simulink model "rmd_power_pack_model"  (R2024a)
settings: Solver=FixedStepAuto  StartTime=0.0  StopTime=10.0  RelTol=1e-3
undefined symbols (not defined in the file): cstCurrSensAmplInpRstn, cstMotorMdlSampTime, cstSpicInvtMdlSampTime, DiscIntNeverNeededParam
libraries: nesl_utility x13, simulink x3, fl_lib x2
(part 1 of 2)
settings Model: DataDictionary=dd_power_pack.sldd  EnableAccessToBaseWorkspace=off  Creator=pav2ofo  LastModifiedBy=pav2ofo

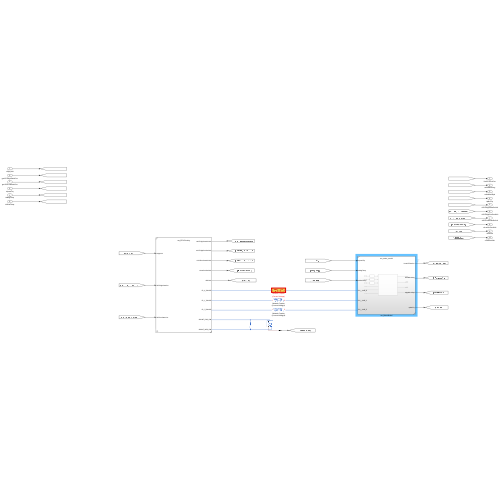
[thumbnail: Simulink's stored preview of the top-level diagram]
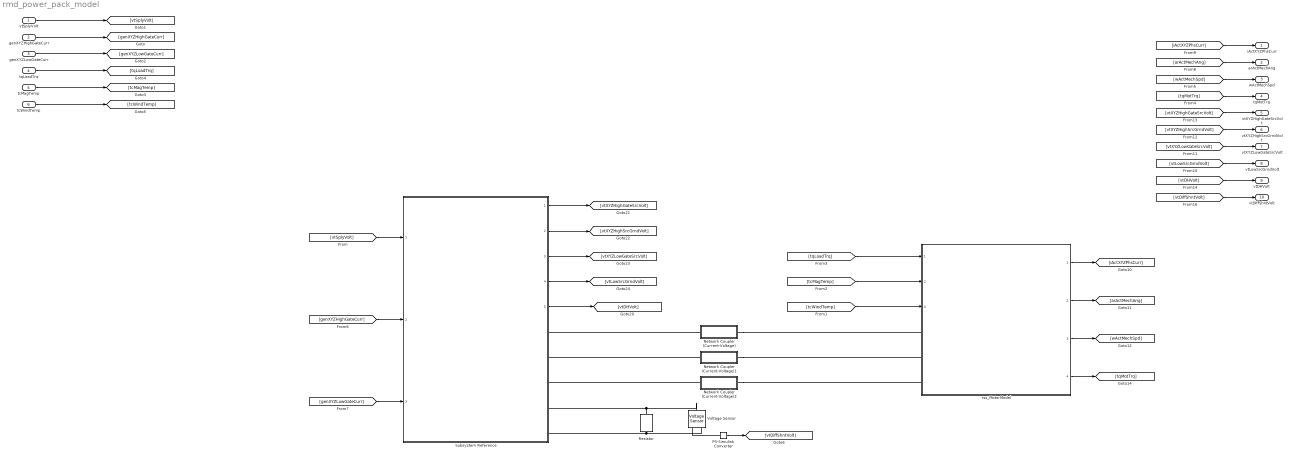
== system rmd_power_pack_model ==
  vtSplyVolt : Inport
  genXYZHighGateCurr : Inport  Port=2
  genXYZLowGateCurr : Inport  Port=3
  tqLoadTrq : Inport  Port=4
  tcMagTemp : Inport  Port=5
  tcWindTemp : Inport  Port=6
  Network Coupler (Current-Voltage) : Subsystem  mask(Network Coupler (Current-Voltage)){}
      mask init:
      | % Icon
      | key = 'Simscape.NetworkCouplers.ElectricalCurrentVoltage';
      | foundation.internal.couplers.updateIcon(gcb,'currentVoltageSource.svg',key)
      settings: OpenFcn=open_system(gcbh,'force')
      mask Help: web([docroot '/simscape/ref/networkcouplercurrentvoltage.html'])
      mask Display:
      | color('red');
      | port_label('LConn', 1,'1')
      | port_label('RConn', 1,'2')
  Network Coupler (Current-Voltage)1 : Subsystem  mask(Network Coupler (Current-Voltage)){}
      mask init:
      | % Icon
      | key = 'Simscape.NetworkCouplers.ElectricalCurrentVoltage';
      | foundation.internal.couplers.updateIcon(gcb,'currentVoltageSource.svg',key)
      settings: OpenFcn=open_system(gcbh,'force')
      mask Help: web([docroot '/simscape/ref/networkcouplercurrentvoltage.html'])
      mask Display:
      | color('red');
      | port_label('LConn', 1,'1')
      | port_label('RConn', 1,'2')
  Network Coupler (Current-Voltage)2 : Subsystem  mask(Network Coupler (Current-Voltage)){}
      mask init:
      | % Icon
      | key = 'Simscape.NetworkCouplers.ElectricalCurrentVoltage';
      | foundation.internal.couplers.updateIcon(gcb,'currentVoltageSource.svg',key)
      settings: OpenFcn=open_system(gcbh,'force')
      mask Help: web([docroot '/simscape/ref/networkcouplercurrentvoltage.html'])
      mask Display:
      | color('red');
      | port_label('LConn', 1,'1')
      | port_label('RConn', 1,'2')
  PS-Simulink Converter : nesl_utility/PS-Simulink Converter  PhysicalDomain=network_engine_domain  SubClassName=ps_output  LeftPortType=input  RightPortType=output  PseudoPeriodic=off  Frequencies=[]  VectorFormat=inherit  Unit=inherit  AffineConversion=off
  Resistor : fl_lib/Electrical/Electrical Elements/Resistor  R=cstCurrSensAmplInpRstn Ohm  i_specify=off  i_priority=None  i=0 A  i_nominal_specify=off  i_nominal_value=1  i_nominal_unit=A  v_specify=off  v_priority=None  v=0 V  v_nominal_specify=off  v_nominal_value=1  v_nominal_unit=V
  Subsystem Reference : Subsystem  SystemSampleTime=cstSpicInvtMdlSampTime  ReferencedSubsystem=rss_ECUCircuitry
  Voltage Sensor : fl_lib/Electrical/Electrical Sensors/Voltage Sensor
  rss_MotorModel : Subsystem  ReferencedSubsystem=rss_motor_model
  iActXYZPhsCurr : Outport
  arActMechAng : Outport  Port=2
  wActMechSpd : Outport  Port=3
  tqMotTrq : Outport  Port=4
  vtXYZHighGateSrcVolt : Outport  Port=5
  vtXYZHighSrcGrndVolt : Outport  Port=6
  vtXYZLowGateSrcVolt : Outport  Port=7
  vtLowSrcGrndVolt : Outport  Port=8
  vtDHVolt : Outport  Port=9
  vtDiffShntVolt : Outport  Port=10
  wires:
  Subsystem Reference/2 -> [vtXYZHighSrcGrndVolt]
  Subsystem Reference/4 -> [vtLowSrcGrndVolt]
  Subsystem Reference/5 -> [vtDHVolt]
  [vtSplyVolt] -> Subsystem Reference/1
  Subsystem Reference/1 -> [vtXYZHighGateSrcVolt]
  Subsystem Reference/3 -> [vtXYZLowGateSrcVolt]
  [genXYZLowGateCurr] -> Subsystem Reference/3
  [tcWindTemp] -> rss_MotorModel/3
  [genXYZHighGateCurr] -> Subsystem Reference/2
  [tqLoadTrq] -> rss_MotorModel/1
  rss_MotorModel/2 -> [arActMechAng]
  rss_MotorModel/4 -> [tqMotTrq]
  rss_MotorModel/3 -> [wActMechSpd]
  rss_MotorModel/1 -> [iActXYZPhsCurr]
  [tcMagTemp] -> rss_MotorModel/2
  vtSplyVolt/1 -> [vtSplyVolt]
  genXYZHighGateCurr/1 -> [genXYZHighGateCurr]
  genXYZLowGateCurr/1 -> [genXYZLowGateCurr]
  tcMagTemp/1 -> [tcMagTemp]
  tcWindTemp/1 -> [tcWindTemp]
  tqLoadTrq/1 -> [tqLoadTrq]
  [arActMechAng] -> arActMechAng/1
  [iActXYZPhsCurr] -> iActXYZPhsCurr/1
  [tqMotTrq] -> tqMotTrq/1
  [wActMechSpd] -> wActMechSpd/1
  [vtXYZLowGateSrcVolt] -> vtXYZLowGateSrcVolt/1
  [vtLowSrcGrndVolt] -> vtLowSrcGrndVolt/1
  [vtXYZHighSrcGrndVolt] -> vtXYZHighSrcGrndVolt/1
  [vtXYZHighGateSrcVolt] -> vtXYZHighGateSrcVolt/1
  [vtDHVolt] -> vtDHVolt/1
  [vtDiffShntVolt] -> vtDiffShntVolt/1
  PS-Simulink Converter/1 -> [vtDiffShntVolt]
  connections:
  Network Coupler (Current-Voltage)1/LConn1 -- Subsystem Reference/RConn2
  Network Coupler (Current-Voltage)/LConn1 -- Subsystem Reference/RConn1
  Network Coupler (Current-Voltage)2/LConn1 -- Subsystem Reference/RConn3
  Network Coupler (Current-Voltage)1/RConn1 -- rss_MotorModel/LConn2
  Network Coupler (Current-Voltage)/RConn1 -- rss_MotorModel/LConn1
  Network Coupler (Current-Voltage)2/RConn1 -- rss_MotorModel/LConn3
  Voltage Sensor/RConn2 -- Resistor/RConn1 -- Subsystem Reference/RConn5
  Resistor/LConn1 -- Voltage Sensor/LConn1 -- Subsystem Reference/RConn4
  PS-Simulink Converter/LConn1 -- Voltage Sensor/RConn1

== system rmd_power_pack_model/Network Coupler (Current-Voltage) ==
  note: Connect Port 1 to the network
      | with the smaller sample time, or
      | the network running variable step.
  note: Uncomment rate transition
      | blocks if one or both networks
      | are running fixed step.
  Port 1 Interface : Subsystem  mask(Network Coupler (Current-Voltage) Port 1 Interface){isThreePhase=off, numNodes=1, samplingType=Fixed step both ports with faster sampling at port 1, ts=1e-3, h1=cstSpicInvtMdlSampTime, h2=cstMotorMdlSampTime, predictionDiscreteToContinuous=off, smoothingContinuousToDiscrete=off, predictionSlowToFast=off, smoothingFastToSlow=off, nSmooth=1, tsSmoothing=0.01, tsMax=0.005, tau=0.001, i0=0, v0=0}
      mask prompts: isThreePhase "physmod:simscape:couplers:SimscapeNetworkCouplersLib:ElectricalThreePhase_MP"; numNodes "physmod:simscape:couplers:SimscapeNetworkCouplersLib:ElectricalNodeArraySize_MP"; samplingType "physmod:simscape:couplers:SimscapeNetworkCouplersLib:SamplingType_MP"; ts "physmod:simscape:couplers:SimscapeNetworkCouplersLib:SeparatorTimeConstants_MP"; h1 "physmod:simscape:couplers:SimscapeNetworkCouplersLib:Port1NetworkDiscreteSampleTimes_MP"; h2 "physmod:simscape:couplers:SimscapeNetworkCouplersLib:Port2NetworkDiscreteSampleTimes_MP"; predictionDiscreteToContinuous "physmod:simscape:couplers:SimscapeNetworkCouplersLib:UsePredictionWhenConnectingFixedStepToVariableStep_MP"; smoothingContinuousToDiscrete "physmod:simscape:couplers:SimscapeNetworkCouplersLib:UseSmoothingWhenConnectingVariableStepToFixedStep_MP"; predictionSlowToFast "physmod:simscape:couplers:SimscapeNetworkCouplersLib:UsePredictionWhenConnectingSlowToFastSampleTimes_MP"; smoothingFastToSlow "physmod:simscape:couplers:SimscapeNetworkCouplersLib:UseSmoothingWhenConnectingFastToSlowSampleTimes_MP"; nSmooth "physmod:simscape:couplers:SimscapeNetworkCouplersLib:NumberOfSamplesOverWhichToSmooth_MP"; tsSmoothing "physmod:simscape:couplers:SimscapeNetworkCouplersLib:SmoothingTimeConstants_MP"; tsMax "physmod:simscape:couplers:SimscapeNetworkCouplersLib:CalculatedFastestTrackableTimeConstants_MP"; tau "physmod:simscape:couplers:SimscapeNetworkCouplersLib:CalculatedFilterTimeConstants_MP"; i0 "physmod:simscape:couplers:SimscapeNetworkCouplersLib:InitialCurrentA_MP"; v0 "physmod:simscape:couplers:SimscapeNetworkCouplersLib:InitialVoltageV_MP"
      mask help: physmod:simscape:couplers:SimscapeNetworkCouplersLib:NetworkCouplerCurrentVoltagePort1Interface_MD
      mask init:
      | % Fixed step sample time value check
      | foundation.internal.couplers.checkSampleTimes(gcb,h1,h2);
      | 
      | % Parameter value checks
      | foundation.internal.couplers.electrical.checkParametersSources(isThreePhase,numNodes,v0,i0);
      | 
      | % Derived parameters
      | [tau,tsMax] = foundation.internal.couplers.electrical.derivedParamsSources(gcb,ts,h1,h2);
      settings: PortSchema="{\"entries\":[{\"content\":{\"sides\":[{\"content\":{\"connectorIds\":[\"LConn1\"]},\"type\":\"ConnectorPlacement.EquallySpacedRectSide\",\"uuid\":\"a6d4a9fd-b5aa-40dc-ab7e-2b646b9b57bc\"},{\"content\":{\"connectorIds\":[\"Out1\",\"In1\"],\"side\":\"RIGHT\"},\"type\":\"ConnectorPlacement.EquallySpacedRectSide\",\"uuid\":\"31bb6273-5b9b-48d0-a1a2-6fbacb979b97\"},{\"content\":{\"connectorIds\":[],\"side\":\"TOP\"},\"type\":\"ConnectorPlacement.EquallySpacedRectSide\",\"uuid\":\"0f7afab2-4481-486c-9ad0-2b42c5b091a4\"}]},\"type\":\"ConnectorPlacement.EquallySpacedConnector\",\"uuid\":\"a98e47aa-cbfd-441a-b14c-c9ea515c056e\"}],\"packageUris\":[\"http://schema.mathworks.com/mf0/Connector/R2020b\"],\"version\":\"1.0\"}"
      mask Help: web([docroot '/simscape/ref/networkcouplercurrentvoltage.html'])
      mask Callback isThreePhase: foundation.internal.couplers.electrical.parameterVisibilitiesThreePhase(gcb)
      mask TypeOptions samplingType: physmod:simscape:couplers:SimscapeNetworkCouplersLib:VariableStepAtPorts1And2_PV | physmod:simscape:couplers:SimscapeNetworkCouplersLib:VariableStepAtPort1AndFixedStepAtPort2_PV | physmod:simscape:couplers:SimscapeNetworkCouplersLib:FixedStepBothPortsWithCommonSampleTime_PV | physmod:simscape:couplers:SimscapeNetworkCouplersLib:FixedStepBothPortsWithFasterSamplingAtPort1_PV
      mask Callback samplingType: foundation.internal.couplers.electrical.parameterVisibilitiesSources(gcb)
      mask Callback predictionDiscreteToContinuous: foundation.internal.couplers.electrical.parameterVisibilitiesSources(gcb)
      mask Callback smoothingContinuousToDiscrete: foundation.internal.couplers.electrical.parameterVisibilitiesSources(gcb)
      mask Callback predictionSlowToFast: foundation.internal.couplers.electrical.parameterVisibilitiesSources(gcb)
      mask Callback smoothingFastToSlow: foundation.internal.couplers.electrical.parameterVisibilitiesSources(gcb)
      mask DialogControl Main Prompt: physmod:simscape:couplers:SimscapeNetworkCouplersLib:tab_Main
      mask DialogControl isThreePhase Prompt: Use three-phase electrical connections
      mask DialogControl numNodes Prompt: Electrical node array size
      mask DialogControl samplingType Prompt: Sampling type
      mask DialogControl ts Prompt: Separator time constant (s)
      mask DialogControl h1 Prompt: Port 1 network discrete sample time (s)
      mask DialogControl h2 Prompt: Port 2 network discrete sample time (s)
      mask DialogControl predictionDiscreteToContinuous Prompt: Use prediction when connecting fixed step to variable step
      mask DialogControl smoothingContinuousToDiscrete Prompt: Use smoothing when connecting variable step to fixed step
      mask DialogControl predictionSlowToFast Prompt: Use prediction when connecting slow to fast sample times
      mask DialogControl smoothingFastToSlow Prompt: Use smoothing when connecting fast to slow sample times
      mask DialogControl nSmooth Prompt: Number of samples over which to smooth
      mask DialogControl tsSmoothing Prompt: Smoothing time constant (s)
      mask DialogControl Analysis Prompt: physmod:simscape:couplers:SimscapeNetworkCouplersLib:tab_Analysis
      mask DialogControl tsMax Prompt: Calculated fastest trackable time constant (s)
      mask DialogControl tau Prompt: Calculated filter time constant (s)
      mask DialogControl updateRecommendations Prompt: physmod:simscape:couplers:SimscapeNetworkCouplersLib:button_Update
      mask DialogControl updateRecommendations Callback: foundation.internal.couplers.electrical.analysisSources(gcb);
      mask DialogControl InitialConditions Prompt: physmod:simscape:couplers:SimscapeNetworkCouplersLib:tab_InitialConditions
      mask DialogControl i0 Prompt: Initial current (A)
      mask DialogControl v0 Prompt: Initial voltage (V)
  Port 2 Interface : Subsystem  mask(Network Coupler (Current-Voltage) Port 2 Interface){isThreePhase=off, numNodes=1}
      mask prompts: isThreePhase "physmod:simscape:couplers:SimscapeNetworkCouplersLib:ElectricalThreePhase_MP"; numNodes "physmod:simscape:couplers:SimscapeNetworkCouplersLib:ElectricalNodeArraySize_MP"
      mask help: physmod:simscape:couplers:SimscapeNetworkCouplersLib:NetworkCouplerCurrentVoltagePort2Interface_MD
      mask init:
      | % Parameter value checks
      | foundation.internal.couplers.electrical.checkParametersNumNodes(isThreePhase,numNodes);
      settings: PortSchema="{\"entries\":[{\"content\":{\"sides\":[{\"content\":{\"connectorIds\":[\"In1\",\"Out1\"]},\"type\":\"ConnectorPlacement.EquallySpacedRectSide\",\"uuid\":\"5a4c1550-e77d-42df-bf3e-b81963920de7\"},{\"content\":{\"connectorIds\":[\"RConn1\"],\"side\":\"RIGHT\"},\"type\":\"ConnectorPlacement.EquallySpacedRectSide\",\"uuid\":\"3fd730f7-5937-4563-a365-595aaae9027b\"},{\"content\":{\"connectorIds\":[],\"side\":\"TOP\"},\"type\":\"ConnectorPlacement.EquallySpacedRectSide\",\"uuid\":\"c16e04e4-26e8-4fd6-98d3-59adbef44c0d\"}]},\"type\":\"ConnectorPlacement.EquallySpacedConnector\",\"uuid\":\"5588d8d0-d459-45fe-a303-1ca6654e99d0\"}],\"packageUris\":[\"http://schema.mathworks.com/mf0/Connector/R2020b\"],\"version\":\"1.0\"}"
      mask Help: web([docroot '/simscape/ref/networkcouplercurrentvoltage.html'])
      mask Callback isThreePhase: foundation.internal.couplers.electrical.parameterVisibilitiesThreePhase(gcb)
      mask DialogControl isThreePhase Prompt: Use three-phase electrical connections
      mask DialogControl numNodes Prompt: Electrical node array size
  Rate transition (fast-to-slow) : RateTransition  Commented=through  Integrity=off
  Rate transition (slow-to-fast) : RateTransition  Commented=through  Integrity=off
  1 : PMIOPort  Side=Left
  2 : PMIOPort  Port=2  Side=Right
  wires:
  Rate transition (slow-to-fast)/1 -> Port 1 Interface/1(current)
  Port 2 Interface/1(current) -> Rate transition (slow-to-fast)/1
  Rate transition (fast-to-slow)/1 -> Port 2 Interface/1(voltage)
  Port 1 Interface/1(voltage) -> Rate transition (fast-to-slow)/1
  connections:
  1/RConn1 -- Port 1 Interface/LConn1
  2/RConn1 -- Port 2 Interface/RConn1

== system rmd_power_pack_model/Network Coupler (Current-Voltage)1 ==
  note: Uncomment rate transition
      | blocks if one or both networks
      | are running fixed step.
  note: Connect Port 1 to the network
      | with the smaller sample time, or
      | the network running variable step.
  Port 1 Interface : Subsystem  mask(Network Coupler (Current-Voltage) Port 1 Interface){isThreePhase=off, numNodes=1, samplingType=Fixed step both ports with faster sampling at port 1, ts=1e-3, h1=10e-9, h2=62.5e-6, predictionDiscreteToContinuous=off, smoothingContinuousToDiscrete=off, predictionSlowToFast=off, smoothingFastToSlow=off, nSmooth=1, tsSmoothing=0.01, tsMax=0.005, tau=0.001, i0=0, v0=0}
      mask prompts: isThreePhase "physmod:simscape:couplers:SimscapeNetworkCouplersLib:ElectricalThreePhase_MP"; numNodes "physmod:simscape:couplers:SimscapeNetworkCouplersLib:ElectricalNodeArraySize_MP"; samplingType "physmod:simscape:couplers:SimscapeNetworkCouplersLib:SamplingType_MP"; ts "physmod:simscape:couplers:SimscapeNetworkCouplersLib:SeparatorTimeConstants_MP"; h1 "physmod:simscape:couplers:SimscapeNetworkCouplersLib:Port1NetworkDiscreteSampleTimes_MP"; h2 "physmod:simscape:couplers:SimscapeNetworkCouplersLib:Port2NetworkDiscreteSampleTimes_MP"; predictionDiscreteToContinuous "physmod:simscape:couplers:SimscapeNetworkCouplersLib:UsePredictionWhenConnectingFixedStepToVariableStep_MP"; smoothingContinuousToDiscrete "physmod:simscape:couplers:SimscapeNetworkCouplersLib:UseSmoothingWhenConnectingVariableStepToFixedStep_MP"; predictionSlowToFast "physmod:simscape:couplers:SimscapeNetworkCouplersLib:UsePredictionWhenConnectingSlowToFastSampleTimes_MP"; smoothingFastToSlow "physmod:simscape:couplers:SimscapeNetworkCouplersLib:UseSmoothingWhenConnectingFastToSlowSampleTimes_MP"; nSmooth "physmod:simscape:couplers:SimscapeNetworkCouplersLib:NumberOfSamplesOverWhichToSmooth_MP"; tsSmoothing "physmod:simscape:couplers:SimscapeNetworkCouplersLib:SmoothingTimeConstants_MP"; tsMax "physmod:simscape:couplers:SimscapeNetworkCouplersLib:CalculatedFastestTrackableTimeConstants_MP"; tau "physmod:simscape:couplers:SimscapeNetworkCouplersLib:CalculatedFilterTimeConstants_MP"; i0 "physmod:simscape:couplers:SimscapeNetworkCouplersLib:InitialCurrentA_MP"; v0 "physmod:simscape:couplers:SimscapeNetworkCouplersLib:InitialVoltageV_MP"
      mask help: physmod:simscape:couplers:SimscapeNetworkCouplersLib:NetworkCouplerCurrentVoltagePort1Interface_MD
      mask init: same as rmd_power_pack_model/Network Coupler (Current-Voltage)/Port 1 Interface
      settings: PortSchema="{\"entries\":[{\"content\":{\"sides\":[{\"content\":{\"connectorIds\":[\"LConn1\"]},\"type\":\"ConnectorPlacement.EquallySpacedRectSide\",\"uuid\":\"a6d4a9fd-b5aa-40dc-ab7e-2b646b9b57bc\"},{\"content\":{\"connectorIds\":[\"Out1\",\"In1\"],\"side\":\"RIGHT\"},\"type\":\"ConnectorPlacement.EquallySpacedRectSide\",\"uuid\":\"31bb6273-5b9b-48d0-a1a2-6fbacb979b97\"},{\"content\":{\"connectorIds\":[],\"side\":\"TOP\"},\"type\":\"ConnectorPlacement.EquallySpacedRectSide\",\"uuid\":\"0f7afab2-4481-486c-9ad0-2b42c5b091a4\"}]},\"type\":\"ConnectorPlacement.EquallySpacedConnector\",\"uuid\":\"a98e47aa-cbfd-441a-b14c-c9ea515c056e\"}],\"packageUris\":[\"http://schema.mathworks.com/mf0/Connector/R2020b\"],\"version\":\"1.0\"}"
      mask Help: web([docroot '/simscape/ref/networkcouplercurrentvoltage.html'])
      mask Callback isThreePhase: foundation.internal.couplers.electrical.parameterVisibilitiesThreePhase(gcb)
      mask TypeOptions samplingType: physmod:simscape:couplers:SimscapeNetworkCouplersLib:VariableStepAtPorts1And2_PV | physmod:simscape:couplers:SimscapeNetworkCouplersLib:VariableStepAtPort1AndFixedStepAtPort2_PV | physmod:simscape:couplers:SimscapeNetworkCouplersLib:FixedStepBothPortsWithCommonSampleTime_PV | physmod:simscape:couplers:SimscapeNetworkCouplersLib:FixedStepBothPortsWithFasterSamplingAtPort1_PV
      mask Callback samplingType: foundation.internal.couplers.electrical.parameterVisibilitiesSources(gcb)
      mask Callback predictionDiscreteToContinuous: foundation.internal.couplers.electrical.parameterVisibilitiesSources(gcb)
      mask Callback smoothingContinuousToDiscrete: foundation.internal.couplers.electrical.parameterVisibilitiesSources(gcb)
      mask Callback predictionSlowToFast: foundation.internal.couplers.electrical.parameterVisibilitiesSources(gcb)
      mask Callback smoothingFastToSlow: foundation.internal.couplers.electrical.parameterVisibilitiesSources(gcb)
      mask DialogControl Main Prompt: physmod:simscape:couplers:SimscapeNetworkCouplersLib:tab_Main
      mask DialogControl isThreePhase Prompt: Use three-phase electrical connections
      mask DialogControl numNodes Prompt: Electrical node array size
      mask DialogControl samplingType Prompt: Sampling type
      mask DialogControl ts Prompt: Separator time constant (s)
      mask DialogControl h1 Prompt: Port 1 network discrete sample time (s)
      mask DialogControl h2 Prompt: Port 2 network discrete sample time (s)
      mask DialogControl predictionDiscreteToContinuous Prompt: Use prediction when connecting fixed step to variable step
      mask DialogControl smoothingContinuousToDiscrete Prompt: Use smoothing when connecting variable step to fixed step
      mask DialogControl predictionSlowToFast Prompt: Use prediction when connecting slow to fast sample times
      mask DialogControl smoothingFastToSlow Prompt: Use smoothing when connecting fast to slow sample times
      mask DialogControl nSmooth Prompt: Number of samples over which to smooth
      mask DialogControl tsSmoothing Prompt: Smoothing time constant (s)
      mask DialogControl Analysis Prompt: physmod:simscape:couplers:SimscapeNetworkCouplersLib:tab_Analysis
      mask DialogControl tsMax Prompt: Calculated fastest trackable time constant (s)
      mask DialogControl tau Prompt: Calculated filter time constant (s)
      mask DialogControl updateRecommendations Prompt: physmod:simscape:couplers:SimscapeNetworkCouplersLib:button_Update
      mask DialogControl updateRecommendations Callback: foundation.internal.couplers.electrical.analysisSources(gcb);
      mask DialogControl InitialConditions Prompt: physmod:simscape:couplers:SimscapeNetworkCouplersLib:tab_InitialConditions
      mask DialogControl i0 Prompt: Initial current (A)
      mask DialogControl v0 Prompt: Initial voltage (V)
  Port 2 Interface : Subsystem  mask(Network Coupler (Current-Voltage) Port 2 Interface){isThreePhase=off, numNodes=1}
      mask prompts: isThreePhase "physmod:simscape:couplers:SimscapeNetworkCouplersLib:ElectricalThreePhase_MP"; numNodes "physmod:simscape:couplers:SimscapeNetworkCouplersLib:ElectricalNodeArraySize_MP"
      mask help: physmod:simscape:couplers:SimscapeNetworkCouplersLib:NetworkCouplerCurrentVoltagePort2Interface_MD
      mask init:
      | % Parameter value checks
      | foundation.internal.couplers.electrical.checkParametersNumNodes(isThreePhase,numNodes);
      settings: PortSchema="{\"entries\":[{\"content\":{\"sides\":[{\"content\":{\"connectorIds\":[\"In1\",\"Out1\"]},\"type\":\"ConnectorPlacement.EquallySpacedRectSide\",\"uuid\":\"5a4c1550-e77d-42df-bf3e-b81963920de7\"},{\"content\":{\"connectorIds\":[\"RConn1\"],\"side\":\"RIGHT\"},\"type\":\"ConnectorPlacement.EquallySpacedRectSide\",\"uuid\":\"3fd730f7-5937-4563-a365-595aaae9027b\"},{\"content\":{\"connectorIds\":[],\"side\":\"TOP\"},\"type\":\"ConnectorPlacement.EquallySpacedRectSide\",\"uuid\":\"c16e04e4-26e8-4fd6-98d3-59adbef44c0d\"}]},\"type\":\"ConnectorPlacement.EquallySpacedConnector\",\"uuid\":\"5588d8d0-d459-45fe-a303-1ca6654e99d0\"}],\"packageUris\":[\"http://schema.mathworks.com/mf0/Connector/R2020b\"],\"version\":\"1.0\"}"
      mask Help: web([docroot '/simscape/ref/networkcouplercurrentvoltage.html'])
      mask Callback isThreePhase: foundation.internal.couplers.electrical.parameterVisibilitiesThreePhase(gcb)
      mask DialogControl isThreePhase Prompt: Use three-phase electrical connections
      mask DialogControl numNodes Prompt: Electrical node array size
  Rate transition (fast-to-slow) : RateTransition  Commented=through  Integrity=off
  Rate transition (slow-to-fast) : RateTransition  Commented=through  Integrity=off
  1 : PMIOPort  Side=Left
  2 : PMIOPort  Port=2  Side=Right
  wires:
  Port 1 Interface/1(voltage) -> Rate transition (fast-to-slow)/1
  Rate transition (fast-to-slow)/1 -> Port 2 Interface/1(voltage)
  Port 2 Interface/1(current) -> Rate transition (slow-to-fast)/1
  Rate transition (slow-to-fast)/1 -> Port 1 Interface/1(current)
  connections:
  2/RConn1 -- Port 2 Interface/RConn1
  1/RConn1 -- Port 1 Interface/LConn1

== system rmd_power_pack_model/Network Coupler (Current-Voltage)2 ==
  note: Connect Port 1 to the network
      | with the smaller sample time, or
      | the network running variable step.
  note: Uncomment rate transition
      | blocks if one or both networks
      | are running fixed step.
  Port 1 Interface : Subsystem  mask(Network Coupler (Current-Voltage) Port 1 Interface){isThreePhase=off, numNodes=1, samplingType=Fixed step both ports with faster sampling at port 1, ts=1e-3, h1=10e-9, h2=62.5e-6, predictionDiscreteToContinuous=off, smoothingContinuousToDiscrete=off, predictionSlowToFast=off, smoothingFastToSlow=off, nSmooth=1, tsSmoothing=0.01, tsMax=0.005, tau=0.001, i0=0, v0=0}
      mask prompts: isThreePhase "physmod:simscape:couplers:SimscapeNetworkCouplersLib:ElectricalThreePhase_MP"; numNodes "physmod:simscape:couplers:SimscapeNetworkCouplersLib:ElectricalNodeArraySize_MP"; samplingType "physmod:simscape:couplers:SimscapeNetworkCouplersLib:SamplingType_MP"; ts "physmod:simscape:couplers:SimscapeNetworkCouplersLib:SeparatorTimeConstants_MP"; h1 "physmod:simscape:couplers:SimscapeNetworkCouplersLib:Port1NetworkDiscreteSampleTimes_MP"; h2 "physmod:simscape:couplers:SimscapeNetworkCouplersLib:Port2NetworkDiscreteSampleTimes_MP"; predictionDiscreteToContinuous "physmod:simscape:couplers:SimscapeNetworkCouplersLib:UsePredictionWhenConnectingFixedStepToVariableStep_MP"; smoothingContinuousToDiscrete "physmod:simscape:couplers:SimscapeNetworkCouplersLib:UseSmoothingWhenConnectingVariableStepToFixedStep_MP"; predictionSlowToFast "physmod:simscape:couplers:SimscapeNetworkCouplersLib:UsePredictionWhenConnectingSlowToFastSampleTimes_MP"; smoothingFastToSlow "physmod:simscape:couplers:SimscapeNetworkCouplersLib:UseSmoothingWhenConnectingFastToSlowSampleTimes_MP"; nSmooth "physmod:simscape:couplers:SimscapeNetworkCouplersLib:NumberOfSamplesOverWhichToSmooth_MP"; tsSmoothing "physmod:simscape:couplers:SimscapeNetworkCouplersLib:SmoothingTimeConstants_MP"; tsMax "physmod:simscape:couplers:SimscapeNetworkCouplersLib:CalculatedFastestTrackableTimeConstants_MP"; tau "physmod:simscape:couplers:SimscapeNetworkCouplersLib:CalculatedFilterTimeConstants_MP"; i0 "physmod:simscape:couplers:SimscapeNetworkCouplersLib:InitialCurrentA_MP"; v0 "physmod:simscape:couplers:SimscapeNetworkCouplersLib:InitialVoltageV_MP"
      mask help: physmod:simscape:couplers:SimscapeNetworkCouplersLib:NetworkCouplerCurrentVoltagePort1Interface_MD
      mask init: same as rmd_power_pack_model/Network Coupler (Current-Voltage)/Port 1 Interface
      settings: PortSchema="{\"entries\":[{\"content\":{\"sides\":[{\"content\":{\"connectorIds\":[\"LConn1\"]},\"type\":\"ConnectorPlacement.EquallySpacedRectSide\",\"uuid\":\"a6d4a9fd-b5aa-40dc-ab7e-2b646b9b57bc\"},{\"content\":{\"connectorIds\":[\"Out1\",\"In1\"],\"side\":\"RIGHT\"},\"type\":\"ConnectorPlacement.EquallySpacedRectSide\",\"uuid\":\"31bb6273-5b9b-48d0-a1a2-6fbacb979b97\"},{\"content\":{\"connectorIds\":[],\"side\":\"TOP\"},\"type\":\"ConnectorPlacement.EquallySpacedRectSide\",\"uuid\":\"0f7afab2-4481-486c-9ad0-2b42c5b091a4\"}]},\"type\":\"ConnectorPlacement.EquallySpacedConnector\",\"uuid\":\"a98e47aa-cbfd-441a-b14c-c9ea515c056e\"}],\"packageUris\":[\"http://schema.mathworks.com/mf0/Connector/R2020b\"],\"version\":\"1.0\"}"
      mask Help: web([docroot '/simscape/ref/networkcouplercurrentvoltage.html'])
      mask Callback isThreePhase: foundation.internal.couplers.electrical.parameterVisibilitiesThreePhase(gcb)
      mask TypeOptions samplingType: physmod:simscape:couplers:SimscapeNetworkCouplersLib:VariableStepAtPorts1And2_PV | physmod:simscape:couplers:SimscapeNetworkCouplersLib:VariableStepAtPort1AndFixedStepAtPort2_PV | physmod:simscape:couplers:SimscapeNetworkCouplersLib:FixedStepBothPortsWithCommonSampleTime_PV | physmod:simscape:couplers:SimscapeNetworkCouplersLib:FixedStepBothPortsWithFasterSamplingAtPort1_PV
      mask Callback samplingType: foundation.internal.couplers.electrical.parameterVisibilitiesSources(gcb)
      mask Callback predictionDiscreteToContinuous: foundation.internal.couplers.electrical.parameterVisibilitiesSources(gcb)
      mask Callback smoothingContinuousToDiscrete: foundation.internal.couplers.electrical.parameterVisibilitiesSources(gcb)
      mask Callback predictionSlowToFast: foundation.internal.couplers.electrical.parameterVisibilitiesSources(gcb)
      mask Callback smoothingFastToSlow: foundation.internal.couplers.electrical.parameterVisibilitiesSources(gcb)
      mask DialogControl Main Prompt: physmod:simscape:couplers:SimscapeNetworkCouplersLib:tab_Main
      mask DialogControl isThreePhase Prompt: Use three-phase electrical connections
      mask DialogControl numNodes Prompt: Electrical node array size
      mask DialogControl samplingType Prompt: Sampling type
      mask DialogControl ts Prompt: Separator time constant (s)
      mask DialogControl h1 Prompt: Port 1 network discrete sample time (s)
      mask DialogControl h2 Prompt: Port 2 network discrete sample time (s)
      mask DialogControl predictionDiscreteToContinuous Prompt: Use prediction when connecting fixed step to variable step
      mask DialogControl smoothingContinuousToDiscrete Prompt: Use smoothing when connecting variable step to fixed step
      mask DialogControl predictionSlowToFast Prompt: Use prediction when connecting slow to fast sample times
      mask DialogControl smoothingFastToSlow Prompt: Use smoothing when connecting fast to slow sample times
      mask DialogControl nSmooth Prompt: Number of samples over which to smooth
      mask DialogControl tsSmoothing Prompt: Smoothing time constant (s)
      mask DialogControl Analysis Prompt: physmod:simscape:couplers:SimscapeNetworkCouplersLib:tab_Analysis
      mask DialogControl tsMax Prompt: Calculated fastest trackable time constant (s)
      mask DialogControl tau Prompt: Calculated filter time constant (s)
      mask DialogControl updateRecommendations Prompt: physmod:simscape:couplers:SimscapeNetworkCouplersLib:button_Update
      mask DialogControl updateRecommendations Callback: foundation.internal.couplers.electrical.analysisSources(gcb);
      mask DialogControl InitialConditions Prompt: physmod:simscape:couplers:SimscapeNetworkCouplersLib:tab_InitialConditions
      mask DialogControl i0 Prompt: Initial current (A)
      mask DialogControl v0 Prompt: Initial voltage (V)
  Port 2 Interface : Subsystem  mask(Network Coupler (Current-Voltage) Port 2 Interface){isThreePhase=off, numNodes=1}
      mask prompts: isThreePhase "physmod:simscape:couplers:SimscapeNetworkCouplersLib:ElectricalThreePhase_MP"; numNodes "physmod:simscape:couplers:SimscapeNetworkCouplersLib:ElectricalNodeArraySize_MP"
      mask help: physmod:simscape:couplers:SimscapeNetworkCouplersLib:NetworkCouplerCurrentVoltagePort2Interface_MD
      mask init:
      | % Parameter value checks
      | foundation.internal.couplers.electrical.checkParametersNumNodes(isThreePhase,numNodes);
      settings: PortSchema="{\"entries\":[{\"content\":{\"sides\":[{\"content\":{\"connectorIds\":[\"In1\",\"Out1\"]},\"type\":\"ConnectorPlacement.EquallySpacedRectSide\",\"uuid\":\"5a4c1550-e77d-42df-bf3e-b81963920de7\"},{\"content\":{\"connectorIds\":[\"RConn1\"],\"side\":\"RIGHT\"},\"type\":\"ConnectorPlacement.EquallySpacedRectSide\",\"uuid\":\"3fd730f7-5937-4563-a365-595aaae9027b\"},{\"content\":{\"connectorIds\":[],\"side\":\"TOP\"},\"type\":\"ConnectorPlacement.EquallySpacedRectSide\",\"uuid\":\"c16e04e4-26e8-4fd6-98d3-59adbef44c0d\"}]},\"type\":\"ConnectorPlacement.EquallySpacedConnector\",\"uuid\":\"5588d8d0-d459-45fe-a303-1ca6654e99d0\"}],\"packageUris\":[\"http://schema.mathworks.com/mf0/Connector/R2020b\"],\"version\":\"1.0\"}"
      mask Help: web([docroot '/simscape/ref/networkcouplercurrentvoltage.html'])
      mask Callback isThreePhase: foundation.internal.couplers.electrical.parameterVisibilitiesThreePhase(gcb)
      mask DialogControl isThreePhase Prompt: Use three-phase electrical connections
      mask DialogControl numNodes Prompt: Electrical node array size
  Rate transition (fast-to-slow) : RateTransition  Commented=through  Integrity=off
  Rate transition (slow-to-fast) : RateTransition  Commented=through  Integrity=off
  1 : PMIOPort  Side=Left
  2 : PMIOPort  Port=2  Side=Right
  wires:
  Rate transition (slow-to-fast)/1 -> Port 1 Interface/1(current)
  Port 2 Interface/1(current) -> Rate transition (slow-to-fast)/1
  Rate transition (fast-to-slow)/1 -> Port 2 Interface/1(voltage)
  Port 1 Interface/1(voltage) -> Rate transition (fast-to-slow)/1
  connections:
  1/RConn1 -- Port 1 Interface/LConn1
  2/RConn1 -- Port 2 Interface/RConn1

== system rmd_power_pack_model/Network Coupler (Current-Voltage)/Port 1 Interface ==
  current : Inport
  Controlled Current Source : SimscapeComponentBlock  SourceFile=foundation.internal.couplers.electrical.currentSource  ComponentPath=foundation.internal.couplers.electrical.currentSource  ComponentVariants="[\"foundation.internal.couplers.electrical.currentSource\"]"  ComponentVariantNames="[\"currentSource\"]"  ClassName=currentSource  SchemaVersion=1  threePhase=false  numNodes=numNodes
      settings: CopyFcn=simscape.engine.sli.internal.componentblockcallback(gcbh,'COPY')  PreCopyFcn=simscape.engine.sli.internal.componentblockcallback(gcbh,'PRECOPY')  PreDeleteFcn=simscape.engine.sli.internal.componentblockcallback(gcbh,'PREDELETE')  InternalSimscapePortConfiguration="{\"Bottom\":[],\"Left\":[{\"id\":\"head\",\"label\":\"\",\"type\":\"foundation.electrical.electrical\"}],\"Right\":[{\"id\":\"iT\",\"label\":\"\",\"type\":\"input\"},{\"id\":\"tail\",\"label\":\"\",\"type\":\"foundation.electrical.electrical\"}],\"Top\":[]}"
      mask Type: Controlled Current Source
  Electrical Reference : SimscapeComponentBlock  SourceFile=foundation.internal.couplers.electrical.reference  ComponentPath=foundation.internal.couplers.electrical.reference  ComponentVariants="[\"foundation.internal.couplers.electrical.reference\"]"  ComponentVariantNames="[\"reference\"]"  ClassName=reference  SchemaVersion=1  threePhase=false  numNodes=numNodes
      settings: CopyFcn=simscape.engine.sli.internal.componentblockcallback(gcbh,'COPY')  PreCopyFcn=simscape.engine.sli.internal.componentblockcallback(gcbh,'PRECOPY')  PreDeleteFcn=simscape.engine.sli.internal.componentblockcallback(gcbh,'PREDELETE')  InternalSimscapePortConfiguration="{\"Bottom\":[],\"Left\":[{\"id\":\"p\",\"label\":\"\",\"type\":\"foundation.electrical.electrical\"}],\"Right\":[],\"Top\":[]}"
      mask Type: Electrical Reference
  Electrical Reference1 : SimscapeComponentBlock  SourceFile=foundation.internal.couplers.electrical.reference  ComponentPath=foundation.internal.couplers.electrical.reference  ComponentVariants="[\"foundation.internal.couplers.electrical.reference\"]"  ComponentVariantNames="[\"reference\"]"  ClassName=reference  SchemaVersion=1  threePhase=false  numNodes=numNodes
      settings: CopyFcn=simscape.engine.sli.internal.componentblockcallback(gcbh,'COPY')  PreCopyFcn=simscape.engine.sli.internal.componentblockcallback(gcbh,'PRECOPY')  PreDeleteFcn=simscape.engine.sli.internal.componentblockcallback(gcbh,'PREDELETE')  InternalSimscapePortConfiguration="{\"Bottom\":[],\"Left\":[{\"id\":\"p\",\"label\":\"\",\"type\":\"foundation.electrical.electrical\"}],\"Right\":[],\"Top\":[]}"
      mask Type: Electrical Reference
  Interface : Subsystem  Variant=on  VariantControlMode=label  VariantControl=Variant1  LabelModeActiveChoice=Discrete
      settings: PortSchema="{\"entries\":[{\"content\":{\"sides\":[{\"content\":{\"connectorIds\":[\"In1\",\"Out2\"]},\"type\":\"ConnectorPlacement.EquallySpacedRectSide\",\"uuid\":\"aa56821c-7799-44e3-b228-553c5b43a68d\"},{\"content\":{\"connectorIds\":[\"In2\",\"Out1\"],\"side\":\"RIGHT\"},\"type\":\"ConnectorPlacement.EquallySpacedRectSide\",\"uuid\":\"8658dee5-55e2-4f33-bdec-e6600ce27fc1\"},{\"content\":{\"connectorIds\":[],\"side\":\"TOP\"},\"type\":\"ConnectorPlacement.EquallySpacedRectSide\",\"uuid\":\"2effe9c6-8e61-4f0c-a39b-329d9ffc707d\"}]},\"type\":\"ConnectorPlacement.EquallySpacedConnector\",\"uuid\":\"c8fc8444-dfc7-49a5-9550-b957635f7d8f\"}],\"packageUris\":[\"http://schema.mathworks.com/mf0/Connector/R2020b\"],\"version\":\"1.0\"}"
  Ip : nesl_utility/Simulink-PS Converter  PhysicalDomain=network_engine_domain  SubClassName=ps_input  LeftPortType=input  RightPortType=output  PseudoPeriodic=off  Frequencies=[]  NoiseDistribution=none  NoiseParameters=[]  Unit=A  AffineConversion=off  FilteringAndDerivatives=zero  SimscapeFilterOrder=1  InputFilterTimeConstant=0.001  UdotUserProvided=1
  Voltage Sensor : SimscapeComponentBlock  SourceFile=foundation.internal.couplers.electrical.voltageSensor  ComponentPath=foundation.internal.couplers.electrical.voltageSensor  ComponentVariants="[\"foundation.internal.couplers.electrical.voltageSensor\"]"  ComponentVariantNames="[\"voltageSensor\"]"  ClassName=voltageSensor  SchemaVersion=1  threePhase=false  numNodes=numNodes
      settings: CopyFcn=simscape.engine.sli.internal.componentblockcallback(gcbh,'COPY')  PreCopyFcn=simscape.engine.sli.internal.componentblockcallback(gcbh,'PRECOPY')  PreDeleteFcn=simscape.engine.sli.internal.componentblockcallback(gcbh,'PREDELETE')  InternalSimscapePortConfiguration="{\"Bottom\":[],\"Left\":[{\"id\":\"p\",\"label\":\"+\",\"type\":\"foundation.electrical.electrical\"}],\"Right\":[{\"id\":\"V\",\"label\":\"V\",\"type\":\"output\"},{\"id\":\"n\",\"label\":\"-\",\"type\":\"foundation.electrical.electrical\"}],\"Top\":[]}"
      mask Type: Voltage Sensor
  Vp : nesl_utility/PS-Simulink Converter  PhysicalDomain=network_engine_domain  SubClassName=ps_output  LeftPortType=input  RightPortType=output  PseudoPeriodic=off  Frequencies=[]  VectorFormat=1-D array  Unit=V  AffineConversion=off
  1 : PMIOPort  Side=Left
  voltage : Outport
  wires:
  Interface/2(through1) -> Ip/1
  Vp/1 -> Interface/1(across1)
  current/1 -> Interface/2(through2)
  Interface/1(across2) -> voltage/1
  connections:
  Voltage Sensor/RConn2 -- Electrical Reference1/LConn1
  Controlled Current Source/RConn1 -- Ip/RConn1
  Voltage Sensor/RConn1 -- Vp/LConn1
  Controlled Current Source/LConn1 -- Electrical Reference/LConn1
  Voltage Sensor/LConn1 -- Controlled Current Source/RConn2 -- 1/RConn1

== system rmd_power_pack_model/Network Coupler (Current-Voltage)/Port 2 Interface ==
  voltage : Inport
  Controlled Voltage Source : SimscapeComponentBlock  SourceFile=foundation.internal.couplers.electrical.voltageSource  ComponentPath=foundation.internal.couplers.electrical.voltageSource  ComponentVariants="[\"foundation.internal.couplers.electrical.voltageSource\"]"  ComponentVariantNames="[\"voltageSource\"]"  ClassName=voltageSource  SchemaVersion=1  threePhase=false  numNodes=numNodes
      settings: CopyFcn=simscape.engine.sli.internal.componentblockcallback(gcbh,'COPY')  PreCopyFcn=simscape.engine.sli.internal.componentblockcallback(gcbh,'PRECOPY')  PreDeleteFcn=simscape.engine.sli.internal.componentblockcallback(gcbh,'PREDELETE')  InternalSimscapePortConfiguration="{\"Bottom\":[],\"Left\":[{\"id\":\"p\",\"label\":\"\",\"type\":\"foundation.electrical.electrical\"}],\"Right\":[{\"id\":\"vT\",\"label\":\"\",\"type\":\"input\"},{\"id\":\"n\",\"label\":\"\",\"type\":\"foundation.electrical.electrical\"}],\"Top\":[]}"
      mask Type: Controlled Voltage Source
  Current Sensor : SimscapeComponentBlock  SourceFile=foundation.internal.couplers.electrical.currentSensor  ComponentPath=foundation.internal.couplers.electrical.currentSensor  ComponentVariants="[\"foundation.internal.couplers.electrical.currentSensor\"]"  ComponentVariantNames="[\"currentSensor\"]"  ClassName=currentSensor  SchemaVersion=1  threePhase=false  numNodes=numNodes
      settings: CopyFcn=simscape.engine.sli.internal.componentblockcallback(gcbh,'COPY')  PreCopyFcn=simscape.engine.sli.internal.componentblockcallback(gcbh,'PRECOPY')  PreDeleteFcn=simscape.engine.sli.internal.componentblockcallback(gcbh,'PREDELETE')  InternalSimscapePortConfiguration="{\"Bottom\":[],\"Left\":[{\"id\":\"p\",\"label\":\"+\",\"type\":\"foundation.electrical.electrical\"}],\"Right\":[{\"id\":\"I\",\"label\":\"I\",\"type\":\"output\"},{\"id\":\"n\",\"label\":\"-\",\"type\":\"foundation.electrical.electrical\"}],\"Top\":[]}"
      mask Type: Current Sensor
  Electrical Reference : SimscapeComponentBlock  SourceFile=foundation.internal.couplers.electrical.reference  ComponentPath=foundation.internal.couplers.electrical.reference  ComponentVariants="[\"foundation.internal.couplers.electrical.reference\"]"  ComponentVariantNames="[\"reference\"]"  ClassName=reference  SchemaVersion=1  threePhase=false  numNodes=numNodes
      settings: CopyFcn=simscape.engine.sli.internal.componentblockcallback(gcbh,'COPY')  PreCopyFcn=simscape.engine.sli.internal.componentblockcallback(gcbh,'PRECOPY')  PreDeleteFcn=simscape.engine.sli.internal.componentblockcallback(gcbh,'PREDELETE')  InternalSimscapePortConfiguration="{\"Bottom\":[],\"Left\":[{\"id\":\"p\",\"label\":\"\",\"type\":\"foundation.electrical.electrical\"}],\"Right\":[],\"Top\":[]}"
      mask Type: Electrical Reference
  In : nesl_utility/PS-Simulink Converter  PhysicalDomain=network_engine_domain  SubClassName=ps_output  LeftPortType=input  RightPortType=output  PseudoPeriodic=off  Frequencies=[]  VectorFormat=1-D array  Unit=A  AffineConversion=off
  Vn : nesl_utility/Simulink-PS Converter  PhysicalDomain=network_engine_domain  SubClassName=ps_input  LeftPortType=input  RightPortType=output  PseudoPeriodic=off  Frequencies=[]  NoiseDistribution=none  NoiseParameters=[]  Unit=V  AffineConversion=off  FilteringAndDerivatives=zero  SimscapeFilterOrder=1  InputFilterTimeConstant=0.001  UdotUserProvided=1
  2 : PMIOPort  Side=Right
  current : Outport
  wires:
  voltage/1 -> Vn/1
  In/1 -> current/1
  connections:
  Current Sensor/LConn1 -- 2/RConn1
  Controlled Voltage Source/RConn1 -- Vn/RConn1
  Current Sensor/RConn2 -- Controlled Voltage Source/LConn1
  Controlled Voltage Source/RConn2 -- Electrical Reference/LConn1
  Current Sensor/RConn1 -- In/LConn1

== system rmd_power_pack_model/Network Coupler (Current-Voltage)1/Port 1 Interface ==
  current : Inport
  Controlled Current Source : SimscapeComponentBlock  SourceFile=foundation.internal.couplers.electrical.currentSource  ComponentPath=foundation.internal.couplers.electrical.currentSource  ComponentVariants="[\"foundation.internal.couplers.electrical.currentSource\"]"  ComponentVariantNames="[\"currentSource\"]"  ClassName=currentSource  SchemaVersion=1  threePhase=false  numNodes=numNodes
      settings: CopyFcn=simscape.engine.sli.internal.componentblockcallback(gcbh,'COPY')  PreCopyFcn=simscape.engine.sli.internal.componentblockcallback(gcbh,'PRECOPY')  PreDeleteFcn=simscape.engine.sli.internal.componentblockcallback(gcbh,'PREDELETE')  InternalSimscapePortConfiguration="{\"Bottom\":[],\"Left\":[{\"id\":\"head\",\"label\":\"\",\"type\":\"foundation.electrical.electrical\"}],\"Right\":[{\"id\":\"iT\",\"label\":\"\",\"type\":\"input\"},{\"id\":\"tail\",\"label\":\"\",\"type\":\"foundation.electrical.electrical\"}],\"Top\":[]}"
      mask Type: Controlled Current Source
  Electrical Reference : SimscapeComponentBlock  SourceFile=foundation.internal.couplers.electrical.reference  ComponentPath=foundation.internal.couplers.electrical.reference  ComponentVariants="[\"foundation.internal.couplers.electrical.reference\"]"  ComponentVariantNames="[\"reference\"]"  ClassName=reference  SchemaVersion=1  threePhase=false  numNodes=numNodes
      settings: CopyFcn=simscape.engine.sli.internal.componentblockcallback(gcbh,'COPY')  PreCopyFcn=simscape.engine.sli.internal.componentblockcallback(gcbh,'PRECOPY')  PreDeleteFcn=simscape.engine.sli.internal.componentblockcallback(gcbh,'PREDELETE')  InternalSimscapePortConfiguration="{\"Bottom\":[],\"Left\":[{\"id\":\"p\",\"label\":\"\",\"type\":\"foundation.electrical.electrical\"}],\"Right\":[],\"Top\":[]}"
      mask Type: Electrical Reference
  Electrical Reference1 : SimscapeComponentBlock  SourceFile=foundation.internal.couplers.electrical.reference  ComponentPath=foundation.internal.couplers.electrical.reference  ComponentVariants="[\"foundation.internal.couplers.electrical.reference\"]"  ComponentVariantNames="[\"reference\"]"  ClassName=reference  SchemaVersion=1  threePhase=false  numNodes=numNodes
      settings: CopyFcn=simscape.engine.sli.internal.componentblockcallback(gcbh,'COPY')  PreCopyFcn=simscape.engine.sli.internal.componentblockcallback(gcbh,'PRECOPY')  PreDeleteFcn=simscape.engine.sli.internal.componentblockcallback(gcbh,'PREDELETE')  InternalSimscapePortConfiguration="{\"Bottom\":[],\"Left\":[{\"id\":\"p\",\"label\":\"\",\"type\":\"foundation.electrical.electrical\"}],\"Right\":[],\"Top\":[]}"
      mask Type: Electrical Reference
  Interface : Subsystem  Variant=on  VariantControlMode=label  VariantControl=Variant1  LabelModeActiveChoice=Discrete
      settings: PortSchema="{\"entries\":[{\"content\":{\"sides\":[{\"content\":{\"connectorIds\":[\"In1\",\"Out2\"]},\"type\":\"ConnectorPlacement.EquallySpacedRectSide\",\"uuid\":\"aa56821c-7799-44e3-b228-553c5b43a68d\"},{\"content\":{\"connectorIds\":[\"In2\",\"Out1\"],\"side\":\"RIGHT\"},\"type\":\"ConnectorPlacement.EquallySpacedRectSide\",\"uuid\":\"8658dee5-55e2-4f33-bdec-e6600ce27fc1\"},{\"content\":{\"connectorIds\":[],\"side\":\"TOP\"},\"type\":\"ConnectorPlacement.EquallySpacedRectSide\",\"uuid\":\"2effe9c6-8e61-4f0c-a39b-329d9ffc707d\"}]},\"type\":\"ConnectorPlacement.EquallySpacedConnector\",\"uuid\":\"c8fc8444-dfc7-49a5-9550-b957635f7d8f\"}],\"packageUris\":[\"http://schema.mathworks.com/mf0/Connector/R2020b\"],\"version\":\"1.0\"}"
  Ip : nesl_utility/Simulink-PS Converter  PhysicalDomain=network_engine_domain  SubClassName=ps_input  LeftPortType=input  RightPortType=output  PseudoPeriodic=off  Frequencies=[]  NoiseDistribution=none  NoiseParameters=[]  Unit=A  AffineConversion=off  FilteringAndDerivatives=zero  SimscapeFilterOrder=1  InputFilterTimeConstant=0.001  UdotUserProvided=1
  Voltage Sensor : SimscapeComponentBlock  SourceFile=foundation.internal.couplers.electrical.voltageSensor  ComponentPath=foundation.internal.couplers.electrical.voltageSensor  ComponentVariants="[\"foundation.internal.couplers.electrical.voltageSensor\"]"  ComponentVariantNames="[\"voltageSensor\"]"  ClassName=voltageSensor  SchemaVersion=1  threePhase=false  numNodes=numNodes
      settings: CopyFcn=simscape.engine.sli.internal.componentblockcallback(gcbh,'COPY')  PreCopyFcn=simscape.engine.sli.internal.componentblockcallback(gcbh,'PRECOPY')  PreDeleteFcn=simscape.engine.sli.internal.componentblockcallback(gcbh,'PREDELETE')  InternalSimscapePortConfiguration="{\"Bottom\":[],\"Left\":[{\"id\":\"p\",\"label\":\"+\",\"type\":\"foundation.electrical.electrical\"}],\"Right\":[{\"id\":\"V\",\"label\":\"V\",\"type\":\"output\"},{\"id\":\"n\",\"label\":\"-\",\"type\":\"foundation.electrical.electrical\"}],\"Top\":[]}"
      mask Type: Voltage Sensor
  Vp : nesl_utility/PS-Simulink Converter  PhysicalDomain=network_engine_domain  SubClassName=ps_output  LeftPortType=input  RightPortType=output  PseudoPeriodic=off  Frequencies=[]  VectorFormat=1-D array  Unit=V  AffineConversion=off
  1 : PMIOPort  Side=Left
  voltage : Outport
  wires:
  Interface/1(across2) -> voltage/1
  current/1 -> Interface/2(through2)
  Vp/1 -> Interface/1(across1)
  Interface/2(through1) -> Ip/1
  connections:
  1/RConn1 -- Controlled Current Source/RConn2 -- Voltage Sensor/LConn1
  Controlled Current Source/LConn1 -- Electrical Reference/LConn1
  Voltage Sensor/RConn1 -- Vp/LConn1
  Controlled Current Source/RConn1 -- Ip/RConn1
  Voltage Sensor/RConn2 -- Electrical Reference1/LConn1
